simulink model "Motor_Test"  (R2023b)
settings: Solver=VariableStepAuto  StartTime=0.0  StopTime=10.0  RelTol=1e-3
values from neighbouring files (symbols this model uses):
  b = 0.1    [Battery_with_Motor_Mod.m]
  Capacity = 5    [Battery with Motor_Mod.m]    (also in Battery_with_Motor_Mod.m)
  J = 0.01    [Battery_with_Motor_Mod.m]
  L = 0.5    [Battery_with_Motor_Mod.m]
  R = 1    [Battery_with_Motor_Mod.m]
  R_bat = 0.5    [Battery with Motor_Mod.m]    (also in Battery_with_Motor_Mod.m)
settings Model: Creator=mdhel  LastModifiedBy=mdhel

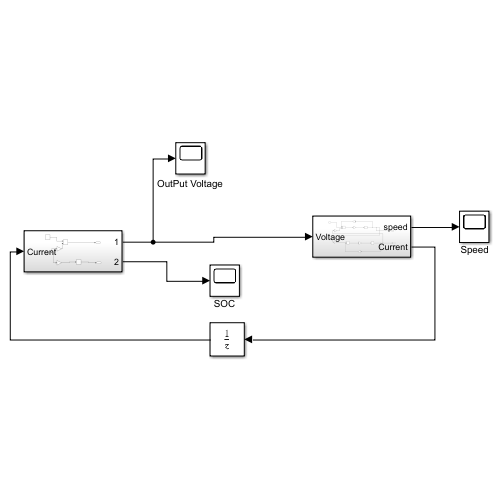
[thumbnail: Simulink's stored preview of the top-level diagram]
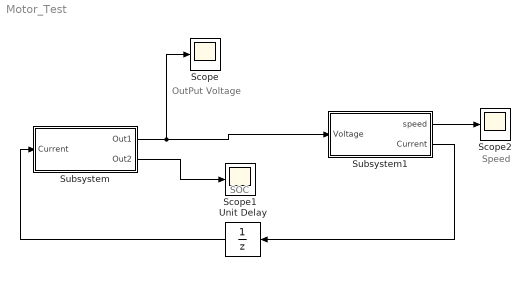
== system Motor_Test ==
  note: OutPut Voltage
  note: SOC
  note: Speed
  Scope : Scope
  Scope1 : Scope
  Scope2 : Scope
  Subsystem : Subsystem
  Subsystem1 : Subsystem
  Unit Delay : UnitDelay  SampleTime=-1  HasFrameUpgradeWarning=on
  wires:
  Subsystem/1(Out1) -> Subsystem1/1(Voltage), Scope/1
  Subsystem/2(Out2) -> Scope1/1
  Subsystem1/1(speed) -> Scope2/1
  Subsystem1/2(Current) -> Unit Delay/1
  Unit Delay/1 -> Subsystem/1(Current)

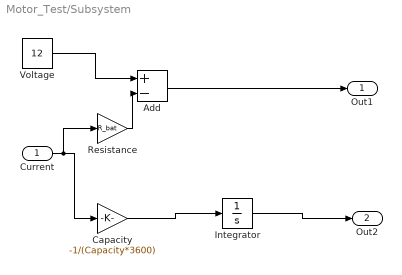
== system Motor_Test/Subsystem ==
  Current : Inport
  Add : Sum  Inputs=+-
  Capacity : Gain  Gain=-1/(Capacity*3600)
  Integrator : Integrator  InitialCondition=1
  Resistance : Gain  Gain=R_bat
  Voltage : Constant  Value=12
  Out1 : Outport
  Out2 : Outport  Port=2
  wires:
  Voltage/1 -> Add/1
  Add/1 -> Out1/1
  Capacity/1 -> Integrator/1
  Integrator/1 -> Out2/1
  Current/1 -> Resistance/1, Capacity/1
  Resistance/1 -> Add/2

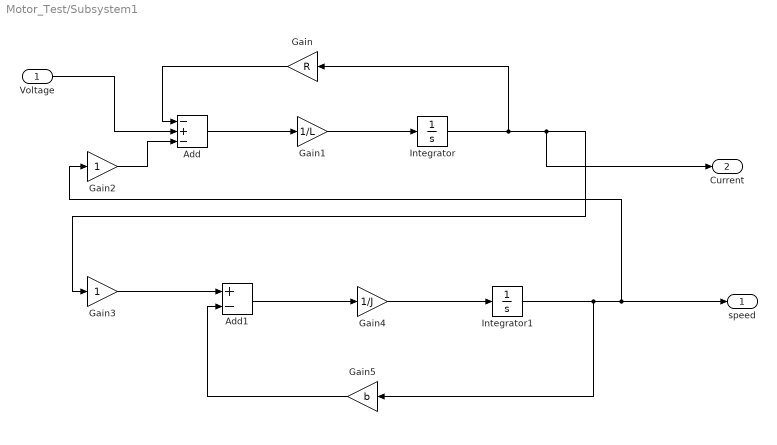
== system Motor_Test/Subsystem1 ==
  Voltage : Inport
  Add : Sum  Inputs=-+-
  Add1 : Sum  Inputs=+-
  Gain : Gain  Gain=R
  Gain1 : Gain  Gain=1/L
  Gain2 : Gain
  Gain3 : Gain
  Gain4 : Gain  Gain=1/J
  Gain5 : Gain  Gain=b
  Integrator : Integrator
  Integrator1 : Integrator
  speed : Outport
  Current : Outport  Port=2
  wires:
  Voltage/1 -> Add/2
  Gain/1 -> Add/1
  Add/1 -> Gain1/1
  Gain1/1 -> Integrator/1
  Integrator/1 -> Gain/1, Current/1, Gain3/1
  Gain2/1 -> Add/3
  Gain3/1 -> Add1/1
  Add1/1 -> Gain4/1
  Gain4/1 -> Integrator1/1
  Integrator1/1 -> Gain5/1, Gain2/1, speed/1
  Gain5/1 -> Add1/2
